simulink model "Movimiento"  (R2023a)
settings: Solver=VariableStepAuto  StartTime=0.0  StopTime=10.0  MaxStep=0.01  RelTol=1e-3
values from neighbouring files (symbols this model uses):
  b1 = 1000    [Mov.m]    (also in Parametros_Mov.m)
  k1 = 16182    [Mov.m]    (also in Parametros_Mov.m)
  k2 = 19000    [Mov.m]    (also in Parametros_Mov.m)
  m1 = 290    [Mov.m]    (also in Parametros_Mov.m)
  m2 = 59    [Mov.m]    (also in Parametros_Mov.m)
libraries: fl_lib x10, nesl_utility x4
settings Model: Creator=PC  LastModifiedBy=webbe
settings OptimizationCC: ReuseModelBlockBuffer=off

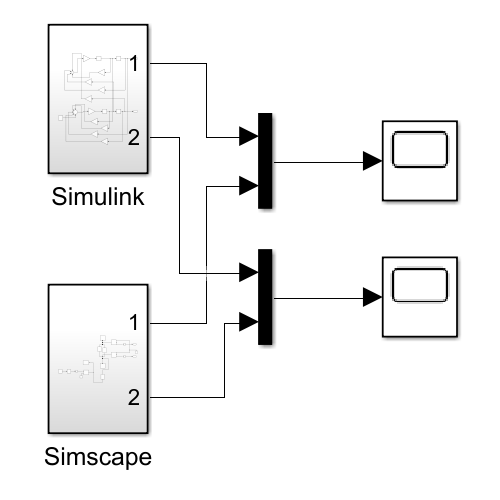
[thumbnail: Simulink's stored preview of the top-level diagram]
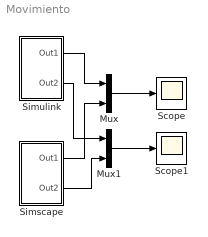
== system Movimiento ==
  Mux : Mux  Inputs=2
  Mux1 : Mux  Inputs=2
  Scope : Scope
  Scope1 : Scope
  Simscape : Subsystem
  Simulink : Subsystem
  wires:
  Simulink/1(Out1) -> Mux/1
  Simscape/1(Out1) -> Mux/2
  Simulink/2(Out2) -> Mux1/1
  Simscape/2(Out2) -> Mux1/2
  Mux/1 -> Scope/1
  Mux1/1 -> Scope1/1

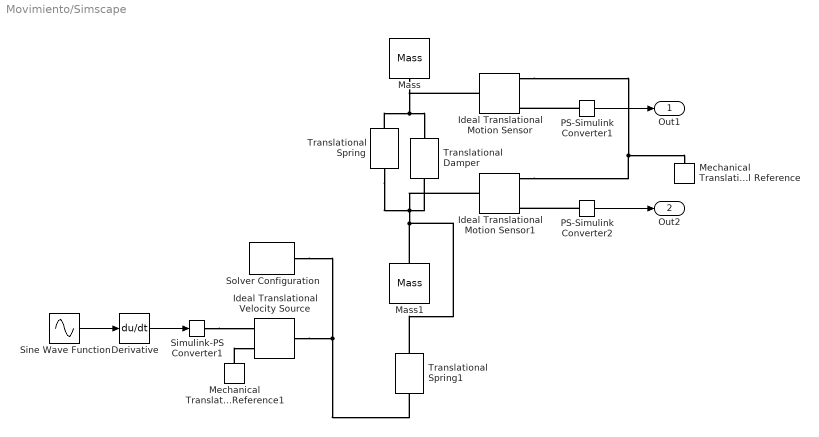
== system Movimiento/Simscape ==
  Derivative : Derivative
  Ideal Translational Motion Sensor : fl_lib/Mechanical/Mechanical Sensors/Ideal Translational Motion Sensor  reference=foundation.enum.MeasurementReference.difference  acceleration_port=false  velocity_port=true  position_port=true  offset=0 m
  Ideal Translational Motion Sensor1 : fl_lib/Mechanical/Mechanical Sensors/Ideal Translational Motion Sensor  reference=foundation.enum.MeasurementReference.difference  acceleration_port=false  velocity_port=true  position_port=true  offset=0 m
  Ideal Translational Velocity Source : fl_lib/Mechanical/Mechanical Sources/Ideal Translational Velocity Source
  Mass : fl_lib/Mechanical/Translational Elements/Mass  mass=m1 kg  num_ports=foundation.enum.numPorts2.one  v_specify=off  v_priority=High  v=0 m/s  v_nominal_specify=off  v_nominal_unit=m/s  v_nominal_value=1  f_specify=off  f_priority=None  f=0 N  f_nominal_specify=off  f_nominal_unit=N  f_nominal_value=1
  Mass1 : fl_lib/Mechanical/Translational Elements/Mass  mass=m2 kg  num_ports=foundation.enum.numPorts2.one  v_specify=off  v_priority=High  v=0 m/s  v_nominal_specify=off  v_nominal_unit=m/s  v_nominal_value=1  f_specify=off  f_priority=None  f=0 N  f_nominal_specify=off  f_nominal_unit=N  f_nominal_value=1
  Mechanical Translational Reference : fl_lib/Mechanical/Translational Elements/Mechanical Translational Reference
  Mechanical Translational Reference1 : fl_lib/Mechanical/Translational Elements/Mechanical Translational Reference
  PS-Simulink Converter1 : nesl_utility/PS-Simulink Converter  PhysicalDomain=network_engine_domain  SubClassName=ps_output  LeftPortType=input  RightPortType=output  PseudoPeriodic=off  Frequencies=[]  VectorFormat=inherit  Unit=inherit  AffineConversion=off
  PS-Simulink Converter2 : nesl_utility/PS-Simulink Converter  PhysicalDomain=network_engine_domain  SubClassName=ps_output  LeftPortType=input  RightPortType=output  PseudoPeriodic=off  Frequencies=[]  VectorFormat=inherit  Unit=inherit  AffineConversion=off
  Simulink-PS Converter1 : nesl_utility/Simulink-PS Converter  PhysicalDomain=network_engine_domain  SubClassName=ps_input  LeftPortType=input  RightPortType=output  PseudoPeriodic=off  Frequencies=[]  NoiseDistribution=none  NoiseParameters=[]  Unit=1  AffineConversion=on  FilteringAndDerivatives=provide  SimscapeFilterOrder=1  InputFilterTimeConstant=0.001  UdotUserProvided=0
  Sine Wave Function : Sin  Amplitude=0.05  Frequency=0.5*pi  SampleTime=0
  Solver Configuration : nesl_utility/Solver Configuration  PhysicalDomain=network_engine_domain  SubClassName=solver  LeftPortType=input  RightPortType=generic  Tones=[]  Harmonics=[]  SimulateNoise=off  Profile=off  UseLocalSampling=off  EnableSwitchedLinearOptims=on  FrequencyDomain=off  UseCCode=off  RelTol=0.001  AbsTol=0.001  MinStep=1e-09  ToWorkspace=off  RevertToSquareIcSolve=off  NumHomotopyIterations=100  PhasorMode=off  PhasorModeNumHarmonics=1  ConsistencySolver=NEWTON_XTOL_AFTER_FTOL  IndexReductionMethod=DerivativeReplacement  DoDC=off  ResidualTolerance=1e-09  ConsistencyTolSource=GLOBAL  ConsistencyAbsTol=0.001  ConsistencyRelTol=0.001  ConsistencyTolFactor=0.001  UseLocalSolver=off  LocalSolverChoice=NE_BACKWARD_EULER_ADVANCER  ResolveIndetEquations=on  FunctionEvalNumThread=1  LocalSolverSampleTime=0.001  DoFixedCost=off  MaxNonlinIter=3  MaxModeIter=2  ComputeImpulses=off  ImpulseIterations=2  LinearAlgebra=auto  LinearAlgebraNumThread=0  EquationFormulation=NE_TIME_EF  DelaysMemoryBudget=1024  AutomaticFiltering=on  FilteringTimeConstant=0.001  PartitionStorageMethod=AS_NEEDED  PartitionMemoryBudget=1024  PartitionMethod=ROBUST
  Translational Damper : fl_lib/Mechanical/Translational Elements/Translational Damper  D=b1 N*s/m  v_specify=off  v_priority=None  v=0 m/s  v_nominal_specify=off  v_nominal_unit=m/s  v_nominal_value=1  f_specify=off  f_priority=None  f=0 N  f_nominal_specify=off  f_nominal_unit=N  f_nominal_value=1
  Translational Spring : fl_lib/Mechanical/Translational Elements/Translational Spring  spr_rate=k1 N/m  v_specify=off  v_priority=None  v=0 m/s  v_nominal_specify=off  v_nominal_unit=m/s  v_nominal_value=1  f_specify=off  f_priority=None  f=0 N  f_nominal_specify=off  f_nominal_unit=N  f_nominal_value=1  x_specify=off  x_priority=High  x=0 m  x_nominal_specify=off  x_nominal_unit=m  x_nominal_value=1
  Translational Spring1 : fl_lib/Mechanical/Translational Elements/Translational Spring  spr_rate=k2 N/m  v_specify=off  v_priority=None  v=0 m/s  v_nominal_specify=off  v_nominal_unit=m/s  v_nominal_value=1  f_specify=off  f_priority=None  f=0 N  f_nominal_specify=off  f_nominal_unit=N  f_nominal_value=1  x_specify=off  x_priority=High  x=0 m  x_nominal_specify=off  x_nominal_unit=m  x_nominal_value=1
  Out1 : Outport
  Out2 : Outport  Port=2
  wires:
  PS-Simulink Converter2/1 -> Out2/1
  Sine Wave Function/1 -> Derivative/1
  Derivative/1 -> Simulink-PS Converter1/1
  PS-Simulink Converter1/1 -> Out1/1
  connections:
  PS-Simulink Converter1/LConn1 -- Ideal Translational Motion Sensor/RConn3
  Translational Spring/LConn1 -- Translational Spring1/RConn1 -- Mass1/LConn1 -- Ideal Translational Motion Sensor1/LConn1 -- Translational Damper/LConn1
  Translational Spring/RConn1 -- Ideal Translational Motion Sensor/LConn1 -- Mass/LConn1 -- Translational Damper/RConn1
  Ideal Translational Motion Sensor1/RConn1 -- Ideal Translational Motion Sensor/RConn1 -- Mechanical Translational Reference/LConn1
  Ideal Translational Velocity Source/LConn1 -- Solver Configuration/RConn1 -- Translational Spring1/LConn1
  Mechanical Translational Reference1/LConn1 -- Ideal Translational Velocity Source/RConn2
  PS-Simulink Converter2/LConn1 -- Ideal Translational Motion Sensor1/RConn3
  Simulink-PS Converter1/RConn1 -- Ideal Translational Velocity Source/RConn1

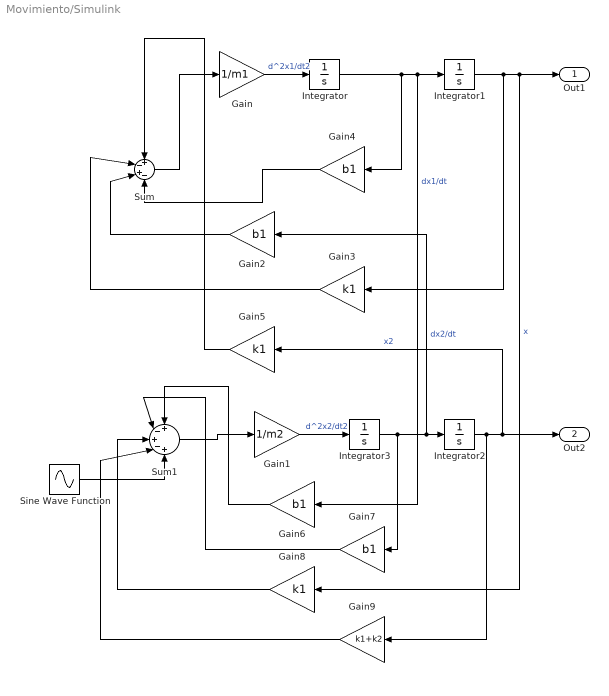
== system Movimiento/Simulink ==
  Gain : Gain  Gain=1/m1
  Gain1 : Gain  Gain=1/m2
  Gain{2,4,6..7} (4 alike) : Gain  Gain=b1
  Gain3 : Gain  Gain=k1
  Gain5 : Gain  Gain=k1
  Gain8 : Gain  Gain=k1
  Gain9 : Gain  Gain=k1+k2
  Integrator{,1..3} (4 alike) : Integrator
  Sine Wave Function : Sin  Amplitude=0.05*k2  Frequency=0.5*pi  SampleTime=0
  Sum : Sum  Inputs=+-+-
  Sum1 : Sum  Inputs=+-+-+
  Out1 : Outport
  Out2 : Outport  Port=2
  wires:
  Integrator1/1 -> Gain3/1, Out1/1, Gain8/1  "x"
  Integrator3/1 -> Gain7/1, Gain2/1, Integrator2/1  "dx2/dt"
  Gain2/1 -> Sum/3
  Gain8/1 -> Sum1/3
  Gain9/1 -> Sum1/4
  Integrator/1 -> Integrator1/1, Gain6/1, Gain4/1  "dx1/dt"
  Gain3/1 -> Sum/2
  Gain7/1 -> Sum1/2
  Integrator2/1 -> Out2/1, Gain5/1, Gain9/1  "x2"
  Sum1/1 -> Gain1/1
  Gain1/1 -> Integrator3/1  "d^2x2/dt2"
  Sum/1 -> Gain/1
  Gain6/1 -> Sum1/1
  Gain/1 -> Integrator/1  "d^2x1/dt2"
  Gain4/1 -> Sum/4
  Gain5/1 -> Sum/1
  Sine Wave Function/1 -> Sum1/5
